simulink model "SystemModel"  (R2020a)
settings: Solver=ode23t  StartTime=0.0  StopTime=inf  RelTol=1e-3
model workspace (MAT data in the model file):
  L = 1
  d = 0.05
settings Model: PacingRate=0.110000  Creator=Mike  LastModifiedBy=Mike

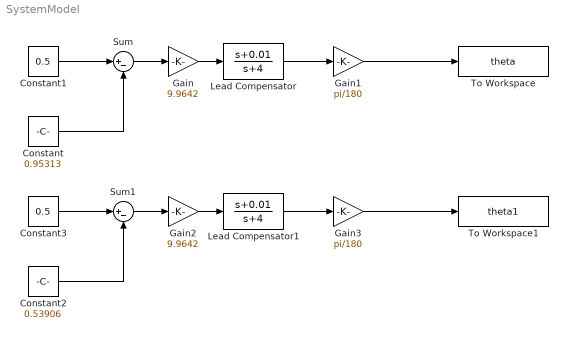
== system SystemModel ==
  Constant : Constant  Value=0.95313
  Constant1 : Constant  Value=0.5
  Constant2 : Constant  Value=0.53906
  Constant3 : Constant  Value=0.5
  Gain : Gain  Gain=9.9642
      settings: AttributesFormatString=%<Gain>
  Gain1 : Gain  Gain=pi/180
      settings: AttributesFormatString=%<Gain>
  Gain2 : Gain  Gain=9.9642
      settings: AttributesFormatString=%<Gain>
  Gain3 : Gain  Gain=pi/180
      settings: AttributesFormatString=%<Gain>
  Lead Compensator : TransferFcn  Numerator=[1 0.01]  Denominator=[1 4]
      settings: AttributesFormatString=|
      | %<Numerator>
      | %<Denominator>
  Lead Compensator1 : TransferFcn  Numerator=[1 0.01]  Denominator=[1 4]
      settings: AttributesFormatString=|
      | %<Numerator>
      | %<Denominator>
  Sum : Sum  Inputs=|+-
  Sum1 : Sum  Inputs=|+-
  To Workspace : ToWorkspace  VariableName=theta  SaveFormat=Timeseries  SampleTime=-1
      settings: MaxDataPoints=1
  To Workspace1 : ToWorkspace  VariableName=theta1  SaveFormat=Timeseries  SampleTime=-1
      settings: MaxDataPoints=1
  wires:
  Lead Compensator/1 -> Gain1/1
  Gain/1 -> Lead Compensator/1
  Constant1/1 -> Sum/1
  Sum/1 -> Gain/1
  Constant/1 -> Sum/2
  Gain1/1 -> To Workspace/1
  Lead Compensator1/1 -> Gain3/1
  Constant3/1 -> Sum1/1
  Gain2/1 -> Lead Compensator1/1
  Constant2/1 -> Sum1/2
  Sum1/1 -> Gain2/1
  Gain3/1 -> To Workspace1/1
